simulink model "Signaling_Model_Test"  (R2020b)
settings: Solver=FixedStepDiscrete  StartTime=0.0  StopTime=10  FixedStep=0.02  RelTol=1e-3  EnableMultiTasking=on
libraries: simulink x1, SignalEditorBlockLib x1
settings Model: DataDictionary=Signaling_Sldd.sldd  Creator=mtarek-a  LastModifiedBy=amohsen2
settings ConfigSet: Description=VLS Standard Config for RH850
settings DataIOCC: LimitDataPoints=on  SaveOutput=off  SignalLogging=off  DSMLogging=off  SaveTime=off  ReturnWorkspaceOutputs=off
settings OptimizationCC: DefaultParameterBehavior=Inlined  UseDivisionForNetSlopeComputation=on  DefaultUnderspecifiedDataType=single  InlineInvariantSignals=on  PassReuseOutputArgsAs=Individual arguments  ActiveStateOutputEnumStorageType=int32  InitFltsAndDblsToZero=on  EfficientFloat2IntCast=on  LifeSpan=inf  SimCompilerOptimization=on  EfficientTunableParamExpr=on
settings DebuggingCC: ConsistencyChecking=warning  SignalInfNanChecking=error  SignalRangeChecking=error  ReadBeforeWriteMsg=EnableAllAsError  WriteAfterWriteMsg=EnableAllAsError  WriteAfterReadMsg=EnableAllAsError  AlgebraicLoopMsg=error  ArtificialAlgebraicLoopMsg=error  SaveWithParameterizedLinksMsg=error  SignalResolutionControl=TryResolveAllWithWarning  BlockPriorityViolationMsg=error  MinStepSizeMsg=error  SolverPrmCheckMsg=warning  InheritedTsInSrcMsg=none  SingleTaskRateTransMsg=error  TasksWithSamePriorityMsg=error  SigSpecEnsureSampleTimeMsg=error  CheckMatrixSingularityMsg=error  IntegerOverflowMsg=error  ParameterOverflowMsg=warning  ParameterUnderflowMsg=error  FixptConstUnderflowMsg=error  FixptConstOverflowMsg=error  FixptConstPrecisionLossMsg=warning  UnderSpecifiedDataTypeMsg=warning  UnnecessaryDatatypeConvMsg=warning  VectorMatrixConversionMsg=warning  SignalLabelMismatchMsg=warning  UnconnectedInputMsg=error  UnconnectedOutputMsg=error  UnconnectedLineMsg=error  SFcnCompatibilityMsg=error  FrameProcessingCompatibilityMsg=warning  UniqueDataStoreMsg=error  BusObjectLabelMismatch=error  RootOutportRequireBusObject=error  AssertControl=DisableAll  ModelReferenceIOMsg=warning  ModelReferenceVersionMismatchMessage=warning  ModelReferenceIOMismatchMessage=warning  UnknownTsInhSupMsg=error  ModelReferenceSymbolNameMessage=error  StateNameClashWarn=warning  StrictBusMsg=ErrorOnBusTreatedAsVector  NonBusSignalsTreatedAsBus=error  SFUnusedDataAndEventsDiag=error  SFInvalidInputDataAccessInChartInitDiag=error  SFTransitionOutsideNaturalParentDiag=error  SFUnreachableExecutionPathDiag=error  SFUndirectedBroadcastEventsDiag=error  SFTransitionActionBeforeConditionDiag=error  SFTemporalDelaySmallerThanSampleTimeDiag=error  SFSelfTransitionDiag=error  SFMachineParentedDataDiag=error  ForceCombineOutputUpdateInSim=on  ArithmeticOperatorsInVariantConditions=warning
settings HardwareCC: ProdBitPerPointer=32  ProdBitPerSizeT=32  ProdBitPerPtrDiffT=32  ProdLargestAtomicInteger=Integer  ProdLargestAtomicFloat=None  ProdWordSize=32  ProdLongLongMode=on  ProdHWDeviceType=Renesas->RH850
settings ModelReferenceCC: EnableRefExpFcnMdlSchedulingChecks=off  EnableParallelModelReferenceBuilds=on  ModelReferenceNumInstancesAllowed=Single  PropagateSignalLabelsOutOfModel=off
settings SFSimCC: SimUserSources=Signal_wrapper.c  SimUseLocalCustomCode=off  SimGenImportedTypeDefs=on  CompileTimeRecursionLimit=0  EnableRuntimeRecursion=off  MATLABDynamicMemAlloc=off  CustomCodeUndefinedFunction=UseInterfaceOnly
settings RTWCC: Description=Embedded Coder  SystemTargetFile=ert.tlc  PackageGeneratedCodeAndArtifacts=on  TemplateMakefile=ert_default_tmf  GenerateReport=on  RTWUseLocalCustomCode=off  RTWUseSimCustomCode=on  CustomSource=Signal_wrapper.c  Toolchain=MinGW64 | gmake (64-bit Windows)  BuildConfiguration=Faster Runs  IncludeHyperlinkInReport=on  LaunchReport=on  PortableWordSizes=on  GenerateTraceInfo=on  GenerateTraceReport=on  GenerateTraceReportSl=on  GenerateTraceReportSf=on  GenerateTraceReportEml=on  GenerateCodeMetricsReport=on
settings CodeAppCC: ForceParamTrailComments=on  IgnoreCustomStorageClasses=off  IgnoreTestpoints=on  MaxIdLength=71  OperatorAnnotations=on  SimulinkDataObjDesc=on  SFDataObjDesc=on  MATLABFcnDesc=on  InsertBlockDesc=on  EnableCustomComments=on
settings ERTTargetCC: TargetLangStandard=C99 (ISO)  UtilityFuncGeneration=Shared location  GenerateSampleERTMain=on  IncludeMdlTerminateFcn=off  SuppressErrorStatus=on  SupportAbsoluteTime=off  PurelyIntegerCode=on  SupportNonFinite=off  SupportComplex=off  RemoveDisableFunc=on  ParenthesesLevel=Maximum  CastingMode=Standards  GenerateSharedConstants=off  GenerateASAP2=on  InlinedParameterPlacement=NonHierarchical  ERTCustomFileTemplate=example_file_process.tlc  EnableSignedLeftShifts=off  EnableSignedRightShifts=off
settings ConfigComp: CovScope=ReferencedModels  CovMetricSettings=dcwe

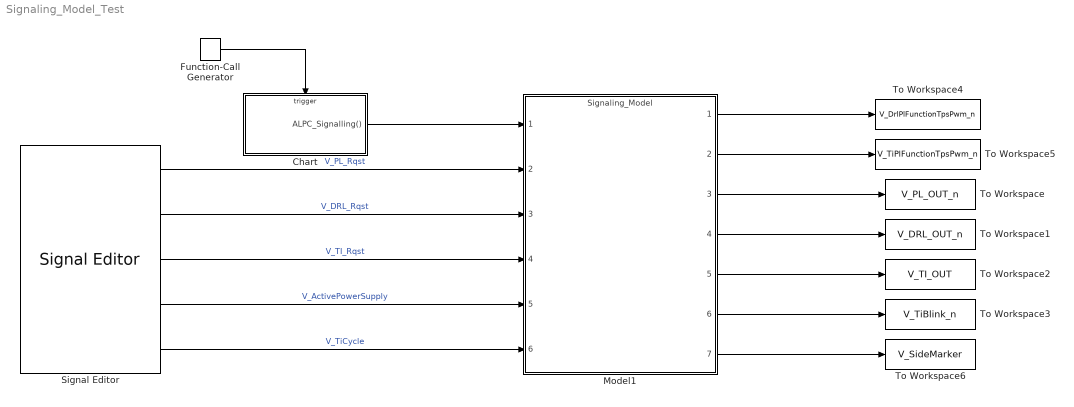
== system Signaling_Model_Test ==
  Chart : Stateflow chart  TreatAsAtomicUnit=on
  Function-Call Generator : simulink/Ports & Subsystems/Function-Call Generator  sample_time=0.02  numberOfIterations=1  DisallowWideOutput=off
  Model1 : ModelReference  ModelNameDialog=Signaling_Model.slx  SimulationMode=Normal  ScheduleRates=on  ModelReferenceVersion=1.136
  Signal Editor : SignalEditorBlockLib/Signal Editor  FileName=C:\E\WS\proj5342_std_signaling\02_TEST\03_INTEGRATION_TESTS\01_TEST_CASES\untitled.mat  ActiveScenario=ID3  ActiveSignal=V_PL_Rqst  IsBus=off  OutputBusObjectStr=Bus: BusObject  SampleTime=0  Interpolate=off  ZeroCross=off  OutputAfterFinalValue=Setting to zero  Unit=inherit  PreserveSignalName=on
  To Workspace : ToWorkspace  VariableName=V_PL_OUT_n  SaveFormat=Timeseries  SampleTime=-1
  To Workspace1 : ToWorkspace  VariableName=V_DRL_OUT_n  SaveFormat=Timeseries  SampleTime=-1
  To Workspace2 : ToWorkspace  VariableName=V_TI_OUT  SaveFormat=Timeseries  SampleTime=-1
  To Workspace3 : ToWorkspace  VariableName=V_TiBlink_n  SaveFormat=Timeseries  SampleTime=-1
  To Workspace4 : ToWorkspace  VariableName=V_DrlPlFunctionTpsPwm_n  SaveFormat=Timeseries  SampleTime=-1
  To Workspace5 : ToWorkspace  VariableName=V_TiPlFunctionTpsPwm_n  SaveFormat=Timeseries  SampleTime=-1
  To Workspace6 : ToWorkspace  VariableName=V_SideMarker  SaveFormat=Timeseries  SampleTime=-1
  wires:
  Signal Editor/3 -> Model1/4  "V_TI_Rqst"
  Function-Call Generator/1 -> Chart/Trigger
  Chart/1(ALPC_Signalling()) -> Model1/1
  Signal Editor/4 -> Model1/5  "V_ActivePowerSupply"
  Model1/1 -> To Workspace4/1
  Model1/2 -> To Workspace5/1
  Signal Editor/5 -> Model1/6  "V_TiCycle"
  Model1/3 -> To Workspace/1
  Model1/4 -> To Workspace1/1
  Signal Editor/1 -> Model1/2  "V_PL_Rqst"
  Signal Editor/2 -> Model1/3  "V_DRL_Rqst"
  Model1/6 -> To Workspace3/1
  Model1/5 -> To Workspace2/1
  Model1/7 -> To Workspace6/1

== stateflow chart Signaling_Model_Test/Chart ==
  settings: executeAtInitialization=1
  state Scheduler
    on every(1,tik):
    send(ALPC_Signalling);
  (default) -> Scheduler
  events: ALPC_Signalling output FUNCTION_CALL_EVENT; tik input FUNCTION_CALL_EVENT
